simulink model "MTTF"  (R2014a)
settings: Solver=ode23t  StartTime=0.0  StopTime=100000000000000  RelTol=1e-3
settings Model: Creator=Divya M  LastModifiedBy=Divya M

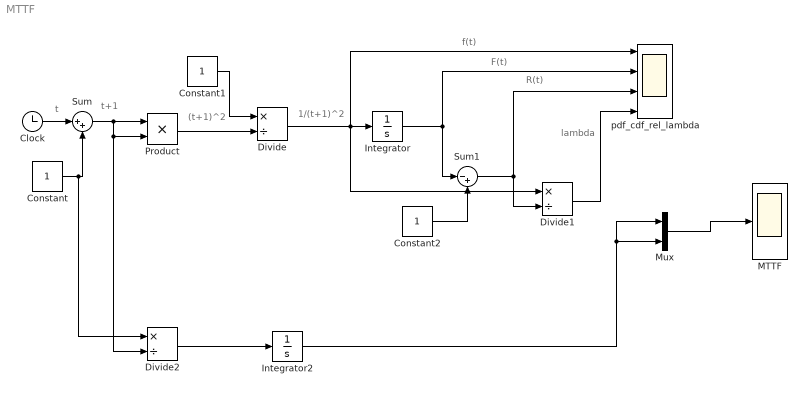
== system MTTF ==
  note: lambda
  note: R(t)
  note: F(t)
  note: f(t)
  note: 1/(t+1)^2
  note: (t+1)^2
  note: t+1
  note: t
  Clock : Clock
  Constant : Constant
  Constant1 : Constant
  Constant2 : Constant
  Divide : Product  Inputs=*/  SaturateOnIntegerOverflow=on  RndMeth=Zero
  Divide1 : Product  Inputs=*/  SaturateOnIntegerOverflow=on  RndMeth=Zero
  Divide2 : Product  Inputs=*/  SaturateOnIntegerOverflow=on  RndMeth=Zero
  Integrator : Integrator
  Integrator2 : Integrator
  MTTF : Scope
      settings: YMin=20  YMax=35  SaveName=ScopeData2
  Mux : Mux  Inputs=2
  Product : Product
  Sum : Sum  Inputs=|++
  Sum1 : Sum  Inputs=|-+
  pdf_cdf_rel_lambda : Scope  NumInputPorts=4
      settings: YMin=-0.1~-0.1~-0.1~-0.1  YMax=1.1~1.1~1.1~1.1
  wires:
  Clock/1 -> Sum/1
  Constant/1 -> Divide2/1, Sum/2
  Product/1 -> Divide/2
  Constant1/1 -> Divide/1
  Divide/1 -> Divide1/1, pdf_cdf_rel_lambda/1, Integrator/1
  Integrator/1 -> Sum1/1, pdf_cdf_rel_lambda/2
  Sum/1 -> Divide2/2, Product/2, Product/1
  Constant2/1 -> Sum1/2
  Sum1/1 -> Divide1/2, pdf_cdf_rel_lambda/3
  Divide1/1 -> pdf_cdf_rel_lambda/4
  Divide2/1 -> Integrator2/1
  Integrator2/1 -> Mux/2, Mux/1
  Mux/1 -> MTTF/1
